simulink model "etc_plant_simple1"  (Simulink 10.1)
settings: Solver=ode45  StartTime=0.0  StopTime=20.0  RelTol=1e-3  EnableMultiTasking=on
model workspace (MAT data in the model file):
  J : num (value not decoded)
settings Model: Creator=cjz  LastModifiedBy=wkmia
settings DataIOCC: ExternalInput=[t,direction,duty]  LimitDataPoints=on  LoadExternalInput=on  SignalLoggingSaveFormat=ModelDataLogs  SaveState=on  DSMLogging=off
settings OptimizationCC: ExpressionDepthLimit=2147483647
settings DebuggingCC: SolverPrmCheckMsg=warning  FcnCallInpInsideContextMsg=warning  StateNameClashWarn=warning

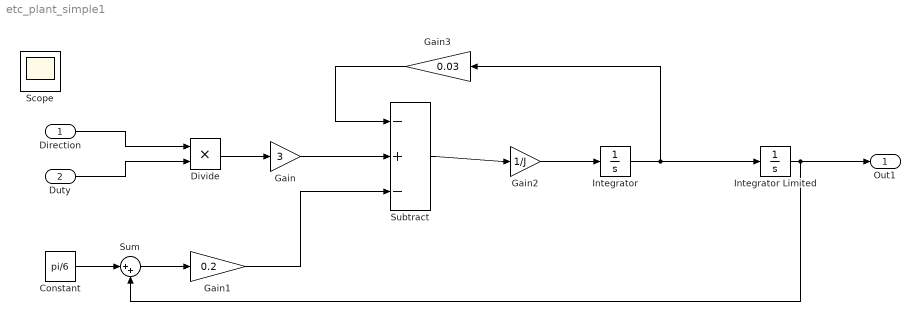
== system etc_plant_simple1 ==
  Direction : Inport
  Duty : Inport  Port=2
  Constant : Constant  Value=pi/6
  Divide : Product  Inputs=**
  Gain : Gain  Gain=3
  Gain1 : Gain  Gain=0.2
  Gain2 : Gain  Gain=1/J
  Gain3 : Gain  Gain=0.03
  Integrator : Integrator
  Integrator Limited : Integrator  InitialCondition=pi/6  LimitOutput=on  UpperSaturationLimit=pi/2  LowerSaturationLimit=0
  Subtract : Sum  Inputs=-+-
  Sum : Sum  Inputs=|++
  Out1 : Outport
  Scope : Scope
  wires:
  Direction/1 -> Divide/1
  Duty/1 -> Divide/2
  Divide/1 -> Gain/1
  Constant/1 -> Sum/1
  Sum/1 -> Gain1/1
  Gain/1 -> Subtract/2
  Gain1/1 -> Subtract/3
  Subtract/1 -> Gain2/1
  Gain2/1 -> Integrator/1
  Integrator/1 -> Integrator Limited/1, Gain3/1
  Gain3/1 -> Subtract/1
  Integrator Limited/1 -> Sum/2, Out1/1
